simulink model "expe1_model_v1"  (R2019b)
settings: Solver=VariableStepAuto  StartTime=0.0  StopTime=time  RelTol=1e-3
values from neighbouring files (symbols this model uses):
  Cs = tf([Kc*tauI Kc],[tauI 0])    [expe1_params_v1.m]
  Fd = tf([Kc*tauD 1], [beta*tauD 1])    [expe1_params_v1.m]
  Gs = tf(1, [1 3 3 1 0])    [expe1_params_v1.m]    (also in expe1_params_v2.m; expe2_params.m = tf([-1 0.4], [1 0.5 0.04]))
  half_time = time/2    (= 25)    [expe1_params_v1.m]    (also in expe1_params_v2.m = 250; expe2_params.m = 50)
  P = Kc    (= 0.56)    [expe1_params_v1.m]    (also in expe1_params_v2.m)
libraries: simulink x1
settings Model: Creator=adityaaaap  LastModifiedBy=adityaaaap

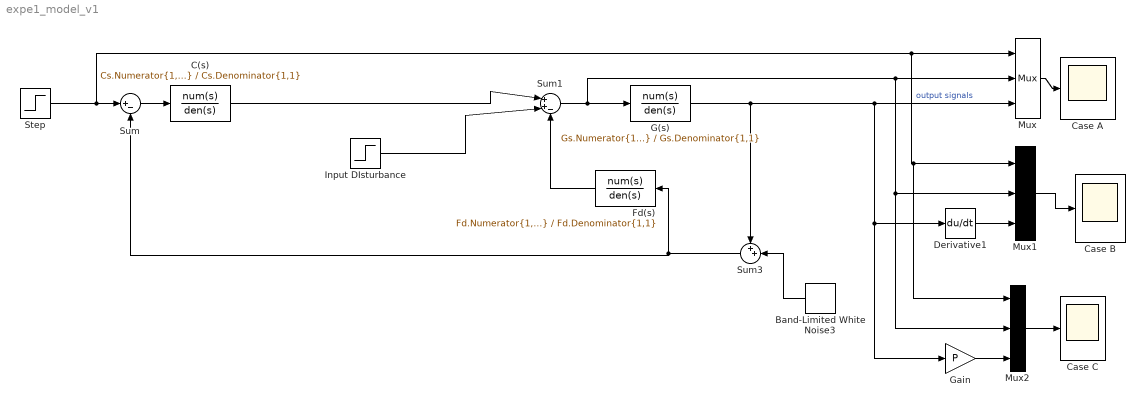
== system expe1_model_v1 ==
  " Fd(s)" : TransferFcn  Numerator=Fd.Numerator{1,1}  Denominator=Fd.Denominator{1,1}
  Band-Limited White Noise3 : simulink/Sources/Band-Limited White Noise  Cov=[0.001]  Ts=0.1  seed=[23341]
  C(s) : TransferFcn  Numerator=Cs.Numerator{1,1}  Denominator=Cs.Denominator{1,1}
  Case A : Scope
  Case B : Scope
  Case C : Scope
  Derivative1 : Derivative
  G(s) : TransferFcn  Numerator=Gs.Numerator{1,1}  Denominator=Gs.Denominator{1,1}
  Gain : Gain  Gain=P
  Input DIsturbance : Step  Time=half_time  After=-3  SampleTime=0
  Mux : Mux  Inputs=3
  Mux1 : Mux  Inputs=3
  Mux2 : Mux  Inputs=3
  Step : Step  Time=0  After=6  SampleTime=0.1
  Sum : Sum  Inputs=|+-
  Sum1 : Sum  Inputs=|++-
  Sum3 : Sum  Inputs=++|
  wires:
  Sum/1 -> C(s)/1
  " Fd(s)"/1 -> Sum1/3
  Mux/1 -> Case A/1
  C(s)/1 -> Sum1/1
  Input DIsturbance/1 -> Sum1/2
  G(s)/1 -> Sum3/1, Derivative1/1, Gain/1, Mux/3  "output signals"
  Sum3/1 -> Sum/2, " Fd(s)"/1
  Sum1/1 -> Mux2/2, Mux1/2, Mux/2, G(s)/1
  Mux1/1 -> Case B/1
  Band-Limited White Noise3/1 -> Sum3/2
  Mux2/1 -> Case C/1
  Step/1 -> Mux2/1, Mux1/1, Mux/1, Sum/1
  Derivative1/1 -> Mux1/3
  Gain/1 -> Mux2/3
